simulink model "chapter4_2021b"  (R2021b)
settings: Solver=VariableStepAuto  StartTime=0.0  StopTime=30  RelTol=1e-3
libraries: Solver_SF x1
settings Model: Creator=CL  LastModifiedBy=CL

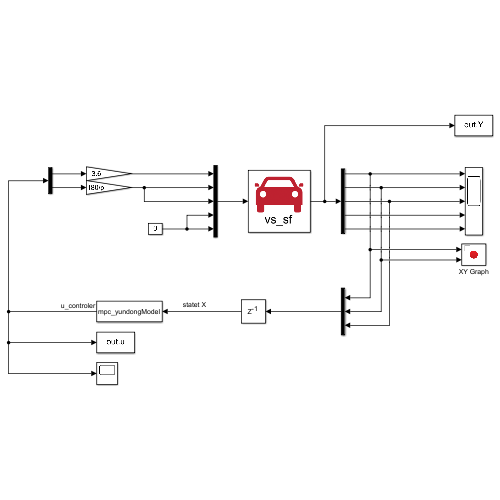
[thumbnail: Simulink's stored preview of the top-level diagram]
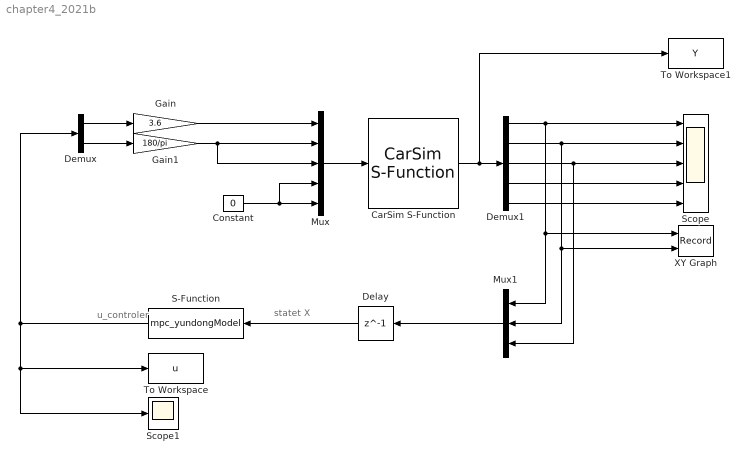
== system chapter4_2021b ==
  note: u_controler
  note: statet X
  CarSim S-Function : Solver_SF/CarSim S-Function  Priority=1  SIMFILE=simfile.sim
  Constant : Constant  Value=0
  Delay : Delay  DelayLength=1  InitialCondition=[0;0;0]
  Demux : Demux  Outputs=2
  Demux1 : Demux  Outputs=5
  Gain : Gain  Gain=3.6
  Gain1 : Gain  Gain=180/pi
  Mux : Mux  Inputs=5
  Mux1 : Mux  Inputs=3
  S-Function : S-Function  FunctionName=mpc_yundongModel  SFunctionDeploymentMode=off  EnableBusSupport=off
  Scope : Scope  NumInputPorts=5
  Scope1 : Scope
  To Workspace : ToWorkspace  VariableName=u  SaveFormat=Timeseries  SampleTime=-1
  To Workspace1 : ToWorkspace  VariableName=Y  SaveFormat=Timeseries  SampleTime=-1
  XY Graph : Record  FileSettingsInternal="{\"entries\":[{\"content\":{\"excelSettings\":{\"content\":{},\"type\":\"Streamout.ExcelSettings\"}},\"type\":\"Streamout.FileSettingStorage\",\"uuid\":\"6b0b94bd-432a-4495-9b81-9143d3b7be01\"}],\"packageUris\":[\"http://schema.mathworks.com/mf0/streamout_blocks/R2020a\"],\"version\":\"1.0\"}"  Layout=[1 1]  SignalsInternal="{\"entries\":[{\"content\":{\"signals\":[{\"content\":{\"blockPath\":[\"chapter4/XY Graph\"],\"channel\":[],\"dimensions\":[1],\"domain\":\"chapter4/XY Graph\",\"lineColor\":\"#a2142f\",\"plots\":[1],\"port\":1,\"sid\":[\"\"],\"signalID\":20,\"signalName\":\"Demux1:1\"},\"type\":\"RecordBlkView.Signal\",\"uuid\":\"073db598-a023-4e4c-8b31-7f54fdc910ee\"},{\"content\":{\"blockPath\":[\"chapter4/XY Graph\"],\"channel\":[],\"dimensions\":[1],\"domain\":\"chapter4/XY Graph\",\"lineColor\":\"#139fff\",\"plots\":[1],\"port\":2,\"sid\":[\"\"],\"signalID\":24,\"signalName\":\"Demux1:2\"},\"type\":\"RecordBlkView.Signal\",\"uuid\":\"985773e9-f57d-410a-97f6-405a58bbb4b5\"}]},\"type\":\"RecordBlkView.InputSignals\",\"uuid\":\"55ea376f-1946-43de-919c-152746f4b74a\"}],\"packageUris\":[\"http://schema.mathworks.com/mf0/streamout_blocks/R2020a\"],\"version\":\"1.0\"}"  VisualizationBindings="{\"xyplotplugin\":{\"info\":[{\"series\":[{\"bindingParametersList\":[{\"parameter\":\"X-Axis\",\"signalID\":20,\"signalName\":\"Demux1:1\"},{\"parameter\":\"Y-Axis\",\"signalID\":24,\"signalName\":\"Demux1:2\"}],\"seriesID\":47687}],\"subplotID\":1}]}}"  CompatibilityTag=XY
  wires:
  Mux/1 -> CarSim S-Function/1
  Demux/1 -> Gain/1
  Demux/2 -> Gain1/1
  S-Function/1 -> Demux/1, To Workspace/1, Scope1/1
  Constant/1 -> Mux/5, Mux/4
  Gain/1 -> Mux/1
  Gain1/1 -> Mux/3, Mux/2
  CarSim S-Function/1 -> To Workspace1/1, Demux1/1
  Mux1/1 -> Delay/1
  Delay/1 -> S-Function/1
  Demux1/1 -> Scope/1, Mux1/1, XY Graph/1
  Demux1/2 -> Scope/2, XY Graph/2, Mux1/2
  Demux1/3 -> Scope/3, Mux1/3
  Demux1/4 -> Scope/4
  Demux1/5 -> Scope/5
